simulink model "w2_warplab_agc"  (Simulink 7.7)
settings: Solver=ode45  StartTime=0.0  StopTime=2e5  RelTol=1e-3
PostLoadFcn:
  | w2_warplab_agc_init
InitFcn:
  | w2_warplab_agc_init
StartFcn:
  | w2_warplab_agc_init
values from neighbouring files (symbols this model uses):
  PHY_CONFIG_PKT_DET_CORR_THRESH = 90    [w2_warplab_agc_init.m]
  PHY_CONFIG_PKT_DET_ENERGY_THRESH = 14    [w2_warplab_agc_init.m]
  PHY_CONFIG_PKT_DET_MIN_DURR = 4    [w2_warplab_agc_init.m]
undefined symbols (not defined in the file or in its folder): gcbh, xlBlockLoadCallback, xlGetNormalizedPeriod
libraries: xbsIndex_r4 x1000, simulink x1
(part 2 of 7)

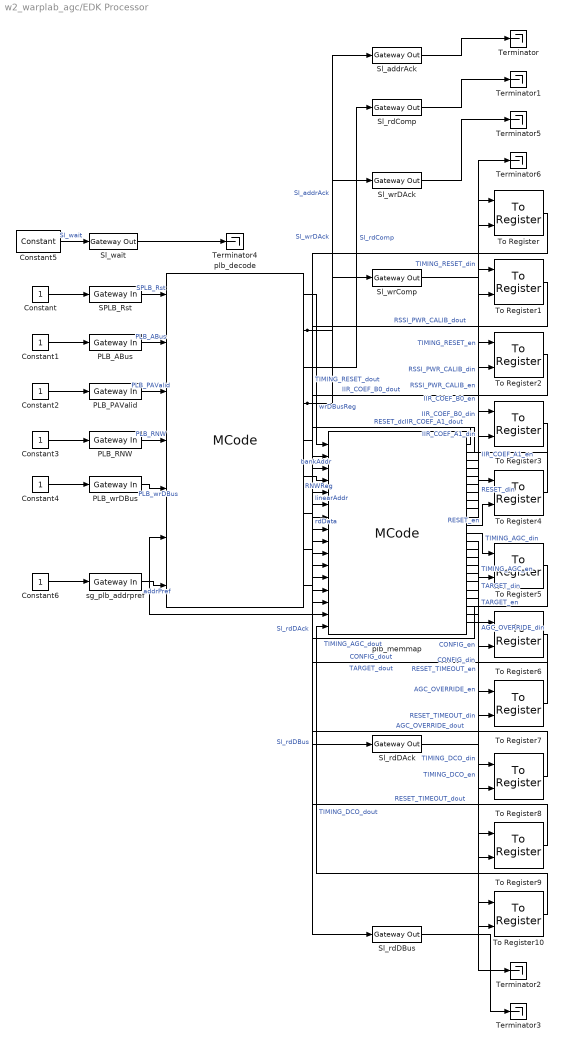
== system w2_warplab_agc/EDK Processor ==
  Constant{,1..4,6} (6 alike) : Constant
  Constant5 : xbsIndex_r4/Constant  const=0  gui_display_data_type=Fixed-point  arith_type=Unsigned  n_bits=1  bin_pt=0  preci_type=Single  exp_width=8  frac_width=24  explicit_period=on  period=xlGetNormalizedPeriod()  equ=P=C  opselect=C  inp2=PCIN>>17  opr=+  inp1=P  carry=CIN  dbl_ovrd=off  block_type=constant
  PLB_ABus : xbsIndex_r4/Gateway In  gui_display_data_type=Fixed-point  arith_type=Unsigned  n_bits=32  bin_pt=0  preci_type=Single  exp_width=8  frac_width=24  quantization="Round  (unbiased: +/- Inf)"  overflow=Saturate  period=xlGetNormalizedPeriod()  dbl_ovrd=off  timing_constraint=None  locs_specified=off  LOCs={}  UseAsADC=off  ADCChannel='1'  inherit_from_input=off  hdl_port=on  block_type=gatewayin
      settings: sginterface={'Xilinx'=>{'jtaghwcosim'=>{'non_memory_mapped_port'=>'PLB_ABus'}},'iopad'=>{'constraint'=>'#'}}
  PLB_PAValid : xbsIndex_r4/Gateway In  gui_display_data_type=Fixed-point  arith_type=Unsigned  n_bits=1  bin_pt=0  preci_type=Single  exp_width=8  frac_width=24  quantization="Round  (unbiased: +/- Inf)"  overflow=Saturate  period=xlGetNormalizedPeriod()  dbl_ovrd=off  timing_constraint=None  locs_specified=off  LOCs={}  UseAsADC=off  ADCChannel='1'  inherit_from_input=off  hdl_port=on  block_type=gatewayin
      settings: sginterface={'Xilinx'=>{'jtaghwcosim'=>{'non_memory_mapped_port'=>'PLB_PAValid'}},'iopad'=>{'constraint'=>'#'}}
  PLB_RNW : xbsIndex_r4/Gateway In  gui_display_data_type=Fixed-point  arith_type=Unsigned  n_bits=1  bin_pt=0  preci_type=Single  exp_width=8  frac_width=24  quantization="Round  (unbiased: +/- Inf)"  overflow=Saturate  period=xlGetNormalizedPeriod()  dbl_ovrd=off  timing_constraint=None  locs_specified=off  LOCs={}  UseAsADC=off  ADCChannel='1'  inherit_from_input=off  hdl_port=on  block_type=gatewayin
      settings: sginterface={'Xilinx'=>{'jtaghwcosim'=>{'non_memory_mapped_port'=>'PLB_RNW'}},'iopad'=>{'constraint'=>'#'}}
  PLB_wrDBus : xbsIndex_r4/Gateway In  gui_display_data_type=Fixed-point  arith_type=Unsigned  n_bits=32  bin_pt=0  preci_type=Single  exp_width=8  frac_width=24  quantization="Round  (unbiased: +/- Inf)"  overflow=Saturate  period=xlGetNormalizedPeriod()  dbl_ovrd=off  timing_constraint=None  locs_specified=off  LOCs={}  UseAsADC=off  ADCChannel='1'  inherit_from_input=off  hdl_port=on  block_type=gatewayin
      settings: sginterface={'Xilinx'=>{'jtaghwcosim'=>{'non_memory_mapped_port'=>'PLB_wrDBus'}},'iopad'=>{'constraint'=>'#'}}
  SPLB_Rst : xbsIndex_r4/Gateway In  gui_display_data_type=Fixed-point  arith_type=Unsigned  n_bits=1  bin_pt=0  preci_type=Single  exp_width=8  frac_width=24  quantization="Round  (unbiased: +/- Inf)"  overflow=Saturate  period=xlGetNormalizedPeriod()  dbl_ovrd=off  timing_constraint=None  locs_specified=off  LOCs={}  UseAsADC=off  ADCChannel='1'  inherit_from_input=off  hdl_port=on  block_type=gatewayin
      settings: sginterface={'Xilinx'=>{'jtaghwcosim'=>{'non_memory_mapped_port'=>'SPLB_Rst'}},'iopad'=>{'constraint'=>'#'}}
  Sl_addrAck : xbsIndex_r4/Gateway Out  inherit_from_input=off  hdl_port=on  timing_constraint=None  locs_specified=off  LOCs={}  UseAsDAC=off  DACChannel='1'  block_type=gatewayout
      settings: sginterface={'Xilinx'=>{'jtaghwcosim'=>{'non_memory_mapped_port'=>'Sl_addrAck'}},'iopad'=>{'constraint'=>'#'}}
  Sl_rdComp : xbsIndex_r4/Gateway Out  inherit_from_input=off  hdl_port=on  timing_constraint=None  locs_specified=off  LOCs={}  UseAsDAC=off  DACChannel='1'  block_type=gatewayout
      settings: sginterface={'Xilinx'=>{'jtaghwcosim'=>{'non_memory_mapped_port'=>'Sl_rdComp'}},'iopad'=>{'constraint'=>'#'}}
  Sl_rdDAck : xbsIndex_r4/Gateway Out  inherit_from_input=off  hdl_port=on  timing_constraint=None  locs_specified=off  LOCs={}  UseAsDAC=off  DACChannel='1'  block_type=gatewayout
      settings: sginterface={'Xilinx'=>{'jtaghwcosim'=>{'non_memory_mapped_port'=>'Sl_rdDAck'}},'iopad'=>{'constraint'=>'#'}}
  Sl_rdDBus : xbsIndex_r4/Gateway Out  inherit_from_input=off  hdl_port=on  timing_constraint=None  locs_specified=off  LOCs={}  UseAsDAC=off  DACChannel='1'  block_type=gatewayout
      settings: sginterface={'Xilinx'=>{'jtaghwcosim'=>{'non_memory_mapped_port'=>'Sl_rdDBus'}},'iopad'=>{'constraint'=>'#'}}
  Sl_wait : xbsIndex_r4/Gateway Out  inherit_from_input=off  hdl_port=on  timing_constraint=None  locs_specified=off  LOCs={}  UseAsDAC=off  DACChannel='1'  block_type=gatewayout
      settings: sginterface={'Xilinx'=>{'jtaghwcosim'=>{'non_memory_mapped_port'=>'Sl_wait'}},'iopad'=>{'constraint'=>'#'}}
  Sl_wrComp : xbsIndex_r4/Gateway Out  inherit_from_input=off  hdl_port=on  timing_constraint=None  locs_specified=off  LOCs={}  UseAsDAC=off  DACChannel='1'  block_type=gatewayout
      settings: sginterface={'Xilinx'=>{'jtaghwcosim'=>{'non_memory_mapped_port'=>'Sl_wrComp'}},'iopad'=>{'constraint'=>'#'}}
  Sl_wrDAck : xbsIndex_r4/Gateway Out  inherit_from_input=off  hdl_port=on  timing_constraint=None  locs_specified=off  LOCs={}  UseAsDAC=off  DACChannel='1'  block_type=gatewayout
      settings: sginterface={'Xilinx'=>{'jtaghwcosim'=>{'non_memory_mapped_port'=>'Sl_wrDAck'}},'iopad'=>{'constraint'=>'#'}}
  Terminator{,1..6} (7 alike) : Terminator
  To Register : xbsIndex_r4/To Register  shared_memory_name='TIMING_RESET'  init=0  ownership=Owned and initialized elsewhere  explicit_data_type=on  gui_display_data_type=Fixed-point  arith_type=Unsigned  n_bits=32  bin_pt=0  preci_type=Single  dbl_ovrd=off  block_type=toreg
      settings: AttributesFormatString=<< %<shared_memory_name> >>  infoedit="Register block that writes data to a shared memory register.  Delay of one sample period."
  To Register1 : xbsIndex_r4/To Register  shared_memory_name='RSSI_PWR_CALIB'  init=0  ownership=Owned and initialized elsewhere  explicit_data_type=on  gui_display_data_type=Fixed-point  arith_type=Unsigned  n_bits=32  bin_pt=0  preci_type=Single  dbl_ovrd=off  block_type=toreg
      settings: AttributesFormatString=<< %<shared_memory_name> >>  infoedit="Register block that writes data to a shared memory register.  Delay of one sample period."
  To Register10 : xbsIndex_r4/To Register  shared_memory_name='TIMING_DCO'  init=0  ownership=Owned and initialized elsewhere  explicit_data_type=on  gui_display_data_type=Fixed-point  arith_type=Unsigned  n_bits=32  bin_pt=0  preci_type=Single  dbl_ovrd=off  block_type=toreg
      settings: AttributesFormatString=<< %<shared_memory_name> >>  infoedit="Register block that writes data to a shared memory register.  Delay of one sample period."
  To Register2 : xbsIndex_r4/To Register  shared_memory_name='IIR_COEF_B0'  init=0  ownership=Owned and initialized elsewhere  explicit_data_type=on  gui_display_data_type=Fixed-point  arith_type=Unsigned  n_bits=18  bin_pt=17  preci_type=Single  dbl_ovrd=off  block_type=toreg
      settings: AttributesFormatString=<< %<shared_memory_name> >>  infoedit="Register block that writes data to a shared memory register.  Delay of one sample period."
  To Register3 : xbsIndex_r4/To Register  shared_memory_name='IIR_COEF_A1'  init=0  ownership=Owned and initialized elsewhere  explicit_data_type=on  gui_display_data_type=Fixed-point  arith_type="Signed  (2's comp)"  n_bits=18  bin_pt=17  preci_type=Single  dbl_ovrd=off  block_type=toreg
      settings: AttributesFormatString=<< %<shared_memory_name> >>  infoedit="Register block that writes data to a shared memory register.  Delay of one sample period."
  To Register4 : xbsIndex_r4/To Register  shared_memory_name='RESET'  init=0  ownership=Owned and initialized elsewhere  explicit_data_type=on  gui_display_data_type=Fixed-point  arith_type=Unsigned  n_bits=32  bin_pt=0  preci_type=Single  dbl_ovrd=off  block_type=toreg
      settings: AttributesFormatString=<< %<shared_memory_name> >>  infoedit="Register block that writes data to a shared memory register.  Delay of one sample period."
  To Register5 : xbsIndex_r4/To Register  shared_memory_name='TIMING_AGC'  init=0  ownership=Owned and initialized elsewhere  explicit_data_type=on  gui_display_data_type=Fixed-point  arith_type=Unsigned  n_bits=32  bin_pt=0  preci_type=Single  dbl_ovrd=off  block_type=toreg
      settings: AttributesFormatString=<< %<shared_memory_name> >>  infoedit="Register block that writes data to a shared memory register.  Delay of one sample period."
  To Register6 : xbsIndex_r4/To Register  shared_memory_name='TARGET'  init=0  ownership=Owned and initialized elsewhere  explicit_data_type=on  gui_display_data_type=Fixed-point  arith_type=Unsigned  n_bits=32  bin_pt=0  preci_type=Single  dbl_ovrd=off  block_type=toreg
      settings: AttributesFormatString=<< %<shared_memory_name> >>  infoedit="Register block that writes data to a shared memory register.  Delay of one sample period."
  To Register7 : xbsIndex_r4/To Register  shared_memory_name='CONFIG'  init=0  ownership=Owned and initialized elsewhere  explicit_data_type=on  gui_display_data_type=Fixed-point  arith_type=Unsigned  n_bits=32  bin_pt=0  preci_type=Single  dbl_ovrd=off  block_type=toreg
      settings: AttributesFormatString=<< %<shared_memory_name> >>  infoedit="Register block that writes data to a shared memory register.  Delay of one sample period."
  To Register8 : xbsIndex_r4/To Register  shared_memory_name='AGC_OVERRIDE'  init=0  ownership=Owned and initialized elsewhere  explicit_data_type=on  gui_display_data_type=Fixed-point  arith_type=Unsigned  n_bits=32  bin_pt=0  preci_type=Single  dbl_ovrd=off  block_type=toreg
      settings: AttributesFormatString=<< %<shared_memory_name> >>  infoedit="Register block that writes data to a shared memory register.  Delay of one sample period."
  To Register9 : xbsIndex_r4/To Register  shared_memory_name='RESET_TIMEOUT'  init=0  ownership=Owned and initialized elsewhere  explicit_data_type=on  gui_display_data_type=Fixed-point  arith_type=Unsigned  n_bits=32  bin_pt=0  preci_type=Single  dbl_ovrd=off  block_type=toreg
      settings: AttributesFormatString=<< %<shared_memory_name> >>  infoedit="Register block that writes data to a shared memory register.  Delay of one sample period."
  plb_decode : xbsIndex_r4/MCode  mfname=xlmax  explicit_period=off  period=1  dbl_ovrd=off  enable_stdout=off  enable_debug=off  mfilecontent=|  suppress_output=on  defparams={}  hide_port_list={}  block_type=mcode
      | function [wrDBusReg, addrAck, rdComp, wrDAck, bankAddr, RNWReg, rdDAck, rdDBus, linearAddr] = plb_bus_decode(plbRst, plbABus, plbPAValid, plbRNW, plbWrDBus, rdData, addrPref)
      | 
      | % constant variables (TODO: should pass from outside)
      | ADDRPREF_LEN = 20;
      | BANKADDR_LEN = 2;
      | LINEARADDR_LEN = 8;
      | ABUS_LEN = 32;
      | DBUS_LEN = 32;
      | 
      | % declare and initialize persistent variables
      | % register input bus signals
      | persistent plbRstReg_, plbRstReg_ = xl_state(0, {xlBoolean});
      | persistent plbABusReg_, plbABusReg_ = xl_state(0, {xlUnsigned, ABUS_LEN, 0});
      | persistent plbPAValidReg_, plbPAValidReg_ = xl_state(0, {xlBoolean});
      | persistent plbRNWReg_, plbRNWReg_ = xl_state(0, {xlUnsigned, 1, 0});
      | persistent plbWrDBusReg_, plbWrDBusReg_ = xl_state(0, {xlUnsigned, DBUS_LEN, 0});
      | 
      | % ===== rest of the outputs =====
      | 
      | bankAddr   = xl_slice(plbABusReg_, 2+BANKADDR_LEN+LINEARADDR_LEN-1, 2+LINEARADDR_LEN);
      | linearAddr = xl_slice(plbABusReg_, 2+LINEARADDR_LEN-1, 2);
      | RNWReg = plbRNWReg_;
      | wrDBusReg = plbWrDBusReg_;
      | 
      | % ===== p_select =====
      | 
      | % register PAValid
      | persistent aValidReg, aValidReg = xl_state(0, {xlBoolean});
      | aValidReg = plbPAValidReg_;
      | 
      | % extract and register the address prefix
      | addrPref_in = xl_slice(plbABusReg_, xl_nbits(plbABusReg_)-1, xl_nbits(plbABusReg_)-ADDRPREF_LEN);
      | if addrPref_in == addrPref
      |     ps1 = true;
      | else 
      |     ps1 = false;
      | end 
      | 
      | persistent ps1Reg, ps1Reg = xl_state(0, ps1);
      | ps1Reg = ps1;
      | 
      | ps = xl_and(ps1Reg, aValidReg);
      | 
      | % ===== addrAck =====
      | 
      | % register ps
      | persistent psReg, psReg = xl_state(0, ps);
      | 
      | addrAck = xfix({xlUnsigned, 1, 0}, xl_and(xl_not(plbRstReg_), ps, xl_not(psReg)));
      | 
      | psReg = ps;
      | 
      | % ===== rdComp, rd/wr DAck =====
      |  
      | rdComp1 = xfix({xlUnsigned, 1, 0}, xl_and(addrAck, RNWReg));
      | 
      | NUM_rdCompDelay = 3;
      | persistent rdCompDelay, rdCompDelay = xl_state(zeros(1, NUM_rdCompDelay), rdComp1, NUM_rdCompDelay);
      | rdComp2 = rdCompDelay.back;
      | rdCompDelay.push_front_pop_back(rdComp1);
      | 
      | persistent rdCompReg, rdCompReg = xl_state(0, rdComp1);
      | rdComp = rdCompReg;
      | rdCompReg = rdComp2;
      | 
      | persistent rdDAckReg, rdDAckReg = xl_state(0, rdComp1);
      | rdDAck = rdDAckReg;
      | rdDAckReg = rdComp;
      | 
      | persistent wrDAckReg, wrDAckReg = xl_state(0, addrAck);
      | wrDAck = wrDAckReg;
      | wrDAckReg = xl_and(addrAck, xl_not(RNWReg));
      | 
      | % ===== rdDBus =====
      | 
      | rdSel = xl_or(rdComp2, rdComp);
      | 
      | if rdSel == 1
      |     rdDBus1 = rdData;
      | else
      |     rdDBus1 = 0;
      | end % if
      | 
      | persistent rdDBusReg, rdDBusReg = xl_state(0, rdDBus1);
      | rdDBus = rdDBusReg;
      | rdDBusReg = rdDBus1;
      | 
      | % rdDBus = xl_concat(rdDBus32, rdDBus32);
      | % rdDBus = rdDBus32;
      | 
      | % ===== update the persistent variables =====
      | 
      | plbRstReg_ = plbRst;
      | plbABusReg_ = plbABus;
      | plbPAValidReg_ = plbPAValid;
      | plbRNWReg_ = plbRNW;
      | plbWrDBusReg_ = xl_slice(plbWrDBus, DBUS_LEN-1, 0);
  plb_memmap : xbsIndex_r4/MCode  mfname=xlmax  explicit_period=off  period=1  dbl_ovrd=off  enable_stdout=off  enable_debug=off  mfilecontent=|  suppress_output=on  defparams={}  hide_port_list={}  block_type=mcode
      | function [read_bank_out, sm_TIMING_RESET_din, sm_TIMING_RESET_en, sm_RSSI_PWR_CALIB_din, sm_RSSI_PWR_CALIB_en, sm_IIR_COEF_B0_din, sm_IIR_COEF_B0_en, sm_IIR_COEF_A1_din, sm_IIR_COEF_A1_en, sm_RESET_din, sm_RESET_en, sm_TIMING_AGC_din, sm_TIMING_AGC_en, sm_TARGET_din, sm_TARGET_en, sm_CONFIG_din, sm_CONFIG_en, sm_AGC_OVERRIDE_din, sm_AGC_OVERRIDE_en, sm_RESET_TIMEOUT_din, sm_RESET_TIMEOUT_en, sm_TIMING_DCO_din, sm_TIMING_DCO_en] = plb_memmap(wrDBus, bankAddr, linearAddr, RNWReg, addrAck, sm_TIMING_RESET, sm_RSSI_PWR_CALIB, sm_IIR_COEF_B0, sm_IIR_COEF_A1, sm_RESET, sm_TIMING_AGC, sm_TARGET, sm_CONFIG, sm_AGC_OVERRIDE, sm_RESET_TIMEOUT, sm_TIMING_DCO)
      | 
      | 
      | % connvert the input data to UFix_32_0 (the bus data type)
      | % 'From Register' blocks
      | % 'To Register' blocks
      | 
      | % sm_TIMING_RESET_dout = xfix({xlUnsigned, 32, 0}, 0);
      | sm_TIMING_RESET_dout = xl_force(sm_TIMING_RESET, xlUnsigned, 0);
      | 
      | % sm_RSSI_PWR_CALIB_dout = xfix({xlUnsigned, 32, 0}, 0);
      | sm_RSSI_PWR_CALIB_dout = xl_force(sm_RSSI_PWR_CALIB, xlUnsigned, 0);
      | 
      | % sm_IIR_COEF_B0_dout = xfix({xlUnsigned, 32, 0}, 0);
      | sm_IIR_COEF_B0_dout = xl_force(sm_IIR_COEF_B0, xlUnsigned, 0);
      | 
      | % sm_IIR_COEF_A1_dout = xfix({xlUnsigned, 32, 0}, 0);
      | sm_IIR_COEF_A1_dout = xl_force(sm_IIR_COEF_A1, xlUnsigned, 0);
      | 
      | % sm_RESET_dout = xfix({xlUnsigned, 32, 0}, 0);
      | sm_RESET_dout = xl_force(sm_RESET, xlUnsigned, 0);
      | 
      | % sm_TIMING_AGC_dout = xfix({xlUnsigned, 32, 0}, 0);
      | sm_TIMING_AGC_dout = xl_force(sm_TIMING_AGC, xlUnsigned, 0);
      | 
      | % sm_TARGET_dout = xfix({xlUnsigned, 32, 0}, 0);
      | sm_TARGET_dout = xl_force(sm_TARGET, xlUnsigned, 0);
      | 
      | % sm_CONFIG_dout = xfix({xlUnsigned, 32, 0}, 0);
      | sm_CONFIG_dout = xl_force(sm_CONFIG, xlUnsigned, 0);
      | 
      | % sm_AGC_OVERRIDE_dout = xfix({xlUnsigned, 32, 0}, 0);
      | sm_AGC_OVERRIDE_dout = xl_force(sm_AGC_OVERRIDE, xlUnsigned, 0);
      | 
      | % sm_RESET_TIMEOUT_dout = xfix({xlUnsigned, 32, 0}, 0);
      | sm_RESET_TIMEOUT_dout = xl_force(sm_RESET_TIMEOUT, xlUnsigned, 0);
      | 
      | % sm_TIMING_DCO_dout = xfix({xlUnsigned, 32, 0}, 0);
      | sm_TIMING_DCO_dout = xl_force(sm_TIMING_DCO, xlUnsigned, 0);
      | 
      | 
      | % 'From FIFO' blocks
      | % 'To FIFO' blocks
      | % 'Shared Memory' blocks
      | 
      | % 'dout' ports of 'From Register' blocks
      | 
      | % registered register mux output
      | persistent reg_bank_out_reg; reg_bank_out_reg = xl_state(0, {xlUnsigned, 32, 0});
      | reg_bank_out = reg_bank_out_reg;
      | 
      | if linearAddr == 0
      |     reg_bank_out_reg = sm_TIMING_RESET_dout;
      | elseif linearAddr == 1
      |     reg_bank_out_reg = sm_RSSI_PWR_CALIB_dout;
      | elseif linearAddr == 2
      |     reg_bank_out_reg = sm_IIR_COEF_B0_dout;
      | elseif linearAddr == 3
      |     reg_bank_out_reg = sm_IIR_COEF_A1_dout;
      | elseif linearAddr == 4
      |     reg_bank_out_reg = sm_RESET_dout;
      | elseif linearAddr == 5
      |     reg_bank_out_reg = sm_TIMING_AGC_dout;
      | elseif linearAddr == 6
      |     reg_bank_out_reg = sm_TARGET_dout;
      | elseif linearAddr == 7
      |     reg_bank_out_reg = sm_CONFIG_dout;
      | elseif linearAddr == 8
      |     reg_bank_out_reg = sm_AGC_OVERRIDE_dout;
      | elseif linearAddr == 9
      |     reg_bank_out_reg = sm_RESET_TIMEOUT_dout;
      | elseif linearAddr == 10
      |     reg_bank_out_reg = sm_TIMING_DCO_dout;
      | 
      | end
      | 
      | 
      | % 'From FIFO' and 'To FIFO' blocks
      | 
      | 
      | 
      | 
      | 
      | opCode = xl_concat(addrAck, RNWReg, bankAddr, linearAddr);
      | 
      | % 'Shared Memory' blocks
      | 
      | 
      | 
      | 
      | 
      | % 'din' ports of 'Shared Memory' blocks
      | 
      | 
      | % 'we' ports of 'Shared Memory' blocks
      | 
      | 
      | % 'addr' ports of 'Shared Memory' blocks
      | 
      | 
      | % 're' ports of 'From FIFO' blocks
      | 
      | 
      | % 'en' ports of 'To Register' blocks
      | if opCode == xl_concat(xfix({xlUnsigned, 4, 0}, 10), ...
      |                        xfix({xlUnsigned, xl_nbits(linearAddr), 0}, 0))
      |     sm_TIMING_RESET_en = true;
      | else
      |     sm_TIMING_RESET_en = false;
      | end
      | if opCode == xl_concat(xfix({xlUnsigned, 4, 0}, 10), ...
      |                        xfix({xlUnsigned, xl_nbits(linearAddr), 0}, 1))
      |     sm_RSSI_PWR_CALIB_en = true;
      | else
      |     sm_RSSI_PWR_CALIB_en = false;
      | end
      | if opCode == xl_concat(xfix({xlUnsigned, 4, 0}, 10), ...
      |                        xfix({xlUnsigned, xl_nbits(linearAddr), 0}, 2))
      |     sm_IIR_COEF_B0_en = true;
      | else
      |     sm_IIR_COEF_B0_en = false;
      | end
      | if opCode == xl_concat(xfix({xlUnsigned, 4, 0}, 10), ...
      |                        xfix({xlUnsigned, xl_nbits(linearAddr), 0}, 3))
      |     sm_IIR_COEF_A1_en = true;
      | else
      |     sm_IIR_COEF_A1_en = false;
      | end
      | if opCode == xl_concat(xfix({xlUnsigned, 4, 0}, 10), ...
      |                        xfix({xlUnsigned, xl_nbits(linearAddr), 0}, 4))
      |     sm_RESET_en = true;
      | else
      |     sm_RESET_en = false;
      | end
      | if opCode == xl_concat(xfix({xlUnsigned, 4, 0}, 10), ...
      |                        xfix({xlUnsigned, xl_nbits(linearAddr), 0}, 5))
      |     sm_TIMING_AGC_en = true;
      | else
      |     sm_TIMING_AGC_en = false;
      | end
      | if opCode == xl_concat(xfix({xlUnsigned, 4, 0}, 10), ...
      |                        xfix({xlUnsigned, xl_nbits(linearAddr), 0}, 6))
      |     sm_TARGET_en = true;
      | else
      |     sm_TARGET_en = false;
      | end
      | if opCode == xl_concat(xfix({xlUnsigned, 4, 0}, 10), ...
      |                        xfix({xlUnsigned, xl_nbits(linearAddr), 0}, 7))
      |     sm_CONFIG_en = true;
      | else
      |     sm_CONFIG_en = false;
      | end
      | if opCode == xl_concat(xfix({xlUnsigned, 4, 0}, 10), ...
      |                        xfix({xlUnsigned, xl_nbits(linearAddr), 0}, 8))
      |     sm_AGC_OVERRIDE_en = true;
      | else
      |     sm_AGC_OVERRIDE_en = false;
      | end
      | if opCode == xl_concat(xfix({xlUnsigned, 4, 0}, 10), ...
      |                        xfix({xlUnsigned, xl_nbits(linearAddr), 0}, 9))
      |     sm_RESET_TIMEOUT_en = true;
      | else
      |     sm_RESET_TIMEOUT_en = false;
      | end
      | if opCode == xl_concat(xfix({xlUnsigned, 4, 0}, 10), ...
      |                        xfix({xlUnsigned, xl_nbits(linearAddr), 0}, 10))
      |     sm_TIMING_DCO_en = true;
      | else
      |     sm_TIMING_DCO_en = false;
      | end
      | 
      | 
      | % 'din' ports of 'To FIFO' blocks
      | 
      | 
      | % 'we' ports of 'To FIFO' blocks
      | 
      | 
      | % 'din' ports of 'To Register' blocks
      | sm_TIMING_RESET_din = xl_force(xl_slice(wrDBus, 32 - 1, 0), ...
      |                                  xlUnsigned, ...
      |                                  0);
      | sm_RSSI_PWR_CALIB_din = xl_force(xl_slice(wrDBus, 32 - 1, 0), ...
      |                                  xlUnsigned, ...
      |                                  0);
      | sm_IIR_COEF_B0_din = xl_force(xl_slice(wrDBus, 18 - 1, 0), ...
      |                                  xlUnsigned, ...
      |                                  17);
      | sm_IIR_COEF_A1_din = xl_force(xl_slice(wrDBus, 18 - 1, 0), ...
      |                                  xlSigned, ...
      |                                  17);
      | sm_RESET_din = xl_force(xl_slice(wrDBus, 32 - 1, 0), ...
      |                                  xlUnsigned, ...
      |                                  0);
      | sm_TIMING_AGC_din = xl_force(xl_slice(wrDBus, 32 - 1, 0), ...
      |                                  xlUnsigned, ...
      |                                  0);
      | sm_TARGET_din = xl_force(xl_slice(wrDBus, 32 - 1, 0), ...
      |                                  xlUnsigned, ...
      |                                  0);
      | sm_CONFIG_din = xl_force(xl_slice(wrDBus, 32 - 1, 0), ...
      |                                  xlUnsigned, ...
      |                                  0);
      | sm_AGC_OVERRIDE_din = xl_force(xl_slice(wrDBus, 32 - 1, 0), ...
      |                                  xlUnsigned, ...
      |                                  0);
      | sm_RESET_TIMEOUT_din = xl_force(xl_slice(wrDBus, 32 - 1, 0), ...
      |                                  xlUnsigned, ...
      |                                  0);
      | sm_TIMING_DCO_din = xl_force(xl_slice(wrDBus, 32 - 1, 0), ...
      |                                  xlUnsigned, ...
      |                                  0);
      | 
      | 
      | persistent read_bank_out_reg; read_bank_out_reg = xl_state(0, {xlUnsigned, 32, 0});
      | read_bank_out = read_bank_out_reg;
      | 
      | persistent bankAddr_reg; bankAddr_reg = xl_state(0, bankAddr);
      | 
      | if bankAddr_reg == 0
      |     % Bank 0: Shared Memories
      |     read_bank_out_reg = 0;
      | elseif bankAddr_reg == 1
      |     % Bank 1: From/To FIFOs
      |     read_bank_out_reg =  0;
      | elseif bankAddr_reg == 2
      |     % Bank 2: From/To Registers
      |     read_bank_out_reg = reg_bank_out;
      | elseif bankAddr_reg == 3
      |     % Bank 3: Configuration Registers
      |     read_bank_out_reg = 0;
      | end
      | 
      | bankAddr_reg = bankAddr;
  sg_plb_addrpref : xbsIndex_r4/Gateway In  gui_display_data_type=Fixed-point  arith_type=Unsigned  n_bits=20  bin_pt=0  preci_type=Single  exp_width=8  frac_width=24  quantization="Round  (unbiased: +/- Inf)"  overflow=Saturate  period=xlGetNormalizedPeriod()  dbl_ovrd=off  timing_constraint=None  locs_specified=off  LOCs={}  UseAsADC=off  ADCChannel='1'  inherit_from_input=off  hdl_port=on  block_type=gatewayin
      settings: sginterface={'Xilinx'=>{'jtaghwcosim'=>{'non_memory_mapped_port'=>'sg_plb_addrpref'}},'iopad'=>{'constraint'=>'#'}}
  wires:
  plb_decode/2 -> plb_memmap/5, Sl_addrAck/1  "Sl_addrAck"
  plb_decode/4 -> Sl_wrDAck/1, Sl_wrComp/1  "Sl_wrDAck"
  plb_memmap/23 -> To Register10/2  "TIMING_DCO_en"
  plb_memmap/22 -> To Register10/1  "TIMING_DCO_din"
  plb_memmap/21 -> To Register9/2  "RESET_TIMEOUT_en"
  plb_memmap/20 -> To Register9/1  "RESET_TIMEOUT_din"
  plb_memmap/19 -> To Register8/2  "AGC_OVERRIDE_en"
  plb_memmap/18 -> To Register8/1  "AGC_OVERRIDE_din"
  plb_memmap/17 -> To Register7/2  "CONFIG_en"
  plb_memmap/16 -> To Register7/1  "CONFIG_din"
  plb_memmap/15 -> To Register6/2  "TARGET_en"
  plb_memmap/14 -> To Register6/1  "TARGET_din"
  plb_memmap/13 -> To Register5/2  "TIMING_AGC_en"
  plb_memmap/12 -> To Register5/1  "TIMING_AGC_din"
  plb_memmap/11 -> To Register4/2  "RESET_en"
  plb_memmap/10 -> To Register4/1  "RESET_din"
  plb_memmap/9 -> To Register3/2  "IIR_COEF_A1_en"
  plb_memmap/8 -> To Register3/1  "IIR_COEF_A1_din"
  plb_memmap/7 -> To Register2/2  "IIR_COEF_B0_en"
  plb_memmap/6 -> To Register2/1  "IIR_COEF_B0_din"
  plb_memmap/5 -> To Register1/2  "RSSI_PWR_CALIB_en"
  plb_memmap/4 -> To Register1/1  "RSSI_PWR_CALIB_din"
  plb_memmap/3 -> To Register/2  "TIMING_RESET_en"
  plb_memmap/2 -> To Register/1  "TIMING_RESET_din"
  plb_memmap/1 -> plb_decode/6  "rdData"
  To Register10/1 -> plb_memmap/16  "TIMING_DCO_dout"
  To Register9/1 -> plb_memmap/15  "RESET_TIMEOUT_dout"
  To Register8/1 -> plb_memmap/14  "AGC_OVERRIDE_dout"
  To Register7/1 -> plb_memmap/13  "CONFIG_dout"
  To Register6/1 -> plb_memmap/12  "TARGET_dout"
  To Register5/1 -> plb_memmap/11  "TIMING_AGC_dout"
  To Register4/1 -> plb_memmap/10  "RESET_dout"
  To Register3/1 -> plb_memmap/9  "IIR_COEF_A1_dout"
  To Register2/1 -> plb_memmap/8  "IIR_COEF_B0_dout"
  To Register1/1 -> plb_memmap/7  "RSSI_PWR_CALIB_dout"
  To Register/1 -> plb_memmap/6  "TIMING_RESET_dout"
  plb_decode/6 -> plb_memmap/4  "RNWReg"
  plb_decode/9 -> plb_memmap/3  "linearAddr"
  plb_decode/5 -> plb_memmap/2  "bankAddr"
  plb_decode/1 -> plb_memmap/1  "wrDBusReg"
  plb_decode/8 -> Sl_rdDBus/1  "Sl_rdDBus"
  plb_decode/7 -> Sl_rdDAck/1  "Sl_rdDAck"
  plb_decode/3 -> Sl_rdComp/1  "Sl_rdComp"
  sg_plb_addrpref/1 -> plb_decode/7  "addrPref"
  PLB_wrDBus/1 -> plb_decode/5  "PLB_wrDBus"
  PLB_RNW/1 -> plb_decode/4  "PLB_RNW"
  PLB_PAValid/1 -> plb_decode/3  "PLB_PAValid"
  PLB_ABus/1 -> plb_decode/2  "PLB_ABus"
  SPLB_Rst/1 -> plb_decode/1  "SPLB_Rst"
  Constant6/1 -> sg_plb_addrpref/1
  Constant5/1 -> Sl_wait/1  "Sl_wait"
  Constant4/1 -> PLB_wrDBus/1
  Constant3/1 -> PLB_RNW/1
  Constant2/1 -> PLB_PAValid/1
  Constant1/1 -> PLB_ABus/1
  Constant/1 -> SPLB_Rst/1
  Sl_wrComp/1 -> Terminator6/1
  Sl_wrDAck/1 -> Terminator5/1
  Sl_wait/1 -> Terminator4/1
  Sl_rdDBus/1 -> Terminator3/1
  Sl_rdDAck/1 -> Terminator2/1
  Sl_rdComp/1 -> Terminator1/1
  Sl_addrAck/1 -> Terminator/1

== system w2_warplab_agc/Gain Calc A ==
  I : Inport
  Q : Inport  Port=2
  IQ Valid : Inport  Port=3
  RSSI : Inport  Port=4
  BB gain : Subsystem
  Capture & Convert : Subsystem
  IQ Mag : Subsystem
  RF Gain : Subsystem
  RSSI Avg : Subsystem
  Register{1..4} (4 alike) : xbsIndex_r4/Register  init=0  rst=off  en=off  dbl_ovrd=off  block_type=register
  G_RF : Outport
  G_BB : Outport  Port=2
  wires:
  RF Gain/1(G_RF) -> Register1/1, Capture & Convert/1(G_RF)
  Register1/1 -> Register2/1
  RSSI/1 -> RSSI Avg/1(RSSI)
  RSSI Avg/1(avg) -> Capture & Convert/2(RSSI)
  Capture & Convert/1(Rx Pwr (dBm)) -> RF Gain/1(Rx Pwr), BB gain/2(P_IN_RSSI)
  Register3/1 -> Register4/1
  BB gain/1(G_BB) -> Register3/1
  RF Gain/2(G_RF_dB) -> BB gain/1(G_RF_dB)
  IQ Mag/1(IQ_dBv) -> BB gain/3(IQ_dBv)
  I/1 -> IQ Mag/1(I)
  Q/1 -> IQ Mag/2(Q)
  IQ Valid/1 -> IQ Mag/3(Valid)
  Register2/1 -> G_RF/1
  Register4/1 -> G_BB/1

== system w2_warplab_agc/Gain Calc B ==
  I : Inport
  Q : Inport  Port=2
  IQ Valid : Inport  Port=3
  RSSI : Inport  Port=4
  BB gain : Subsystem
  Capture & Convert : Subsystem
  IQ Mag : Subsystem
  RF Gain : Subsystem
  RSSI Avg : Subsystem
  Register{1..4} (4 alike) : xbsIndex_r4/Register  init=0  rst=off  en=off  dbl_ovrd=off  block_type=register
  G_RF : Outport
  G_BB : Outport  Port=2
  wires:
  Register4/1 -> G_BB/1
  Register2/1 -> G_RF/1
  IQ Valid/1 -> IQ Mag/3(Valid)
  Q/1 -> IQ Mag/2(Q)
  I/1 -> IQ Mag/1(I)
  IQ Mag/1(IQ_dBv) -> BB gain/3(IQ_dBv)
  RF Gain/2(G_RF_dB) -> BB gain/1(G_RF_dB)
  BB gain/1(G_BB) -> Register3/1
  Register3/1 -> Register4/1
  Capture & Convert/1(Rx Pwr (dBm)) -> BB gain/2(P_IN_RSSI), RF Gain/1(Rx Pwr)
  RSSI Avg/1(avg) -> Capture & Convert/2(RSSI)
  RSSI/1 -> RSSI Avg/1(RSSI)
  Register1/1 -> Register2/1
  RF Gain/1(G_RF) -> Capture & Convert/1(G_RF), Register1/1

== system w2_warplab_agc/Gain Calc C ==
  I : Inport
  Q : Inport  Port=2
  IQ Valid : Inport  Port=3
  RSSI : Inport  Port=4
  BB gain : Subsystem
  Capture & Convert : Subsystem
  IQ Mag : Subsystem
  RF Gain : Subsystem
  RSSI Avg : Subsystem
  Register{1..4} (4 alike) : xbsIndex_r4/Register  init=0  rst=off  en=off  dbl_ovrd=off  block_type=register
  G_RF : Outport
  G_BB : Outport  Port=2
  wires:
  RF Gain/1(G_RF) -> Register1/1, Capture & Convert/1(G_RF)
  Register1/1 -> Register2/1
  RSSI/1 -> RSSI Avg/1(RSSI)
  RSSI Avg/1(avg) -> Capture & Convert/2(RSSI)
  Capture & Convert/1(Rx Pwr (dBm)) -> RF Gain/1(Rx Pwr), BB gain/2(P_IN_RSSI)
  Register3/1 -> Register4/1
  BB gain/1(G_BB) -> Register3/1
  RF Gain/2(G_RF_dB) -> BB gain/1(G_RF_dB)
  IQ Mag/1(IQ_dBv) -> BB gain/3(IQ_dBv)
  I/1 -> IQ Mag/1(I)
  Q/1 -> IQ Mag/2(Q)
  IQ Valid/1 -> IQ Mag/3(Valid)
  Register2/1 -> G_RF/1
  Register4/1 -> G_BB/1

== system w2_warplab_agc/Gain Calc D ==
  I : Inport
  Q : Inport  Port=2
  IQ Valid : Inport  Port=3
  RSSI : Inport  Port=4
  BB gain : Subsystem
  Capture & Convert : Subsystem
  IQ Mag : Subsystem
  RF Gain : Subsystem
  RSSI Avg : Subsystem
  Register{1..4} (4 alike) : xbsIndex_r4/Register  init=0  rst=off  en=off  dbl_ovrd=off  block_type=register
  G_RF : Outport
  G_BB : Outport  Port=2
  wires:
  Register4/1 -> G_BB/1
  Register2/1 -> G_RF/1
  IQ Valid/1 -> IQ Mag/3(Valid)
  Q/1 -> IQ Mag/2(Q)
  I/1 -> IQ Mag/1(I)
  IQ Mag/1(IQ_dBv) -> BB gain/3(IQ_dBv)
  RF Gain/2(G_RF_dB) -> BB gain/1(G_RF_dB)
  BB gain/1(G_BB) -> Register3/1
  Register3/1 -> Register4/1
  Capture & Convert/1(Rx Pwr (dBm)) -> BB gain/2(P_IN_RSSI), RF Gain/1(Rx Pwr)
  RSSI Avg/1(avg) -> Capture & Convert/2(RSSI)
  RSSI/1 -> RSSI Avg/1(RSSI)
  Register1/1 -> Register2/1
  RF Gain/1(G_RF) -> Capture & Convert/1(G_RF), Register1/1

== system w2_warplab_agc/IQ Outputs ==
  IQ Valid : Inport
  A I : Inport  Port=2
  A Q : Inport  Port=3
  B I : Inport  Port=4
  B Q : Inport  Port=5
  C I : Inport  Port=6
  C Q : Inport  Port=7
  D I : Inport  Port=8
  D Q : Inport  Port=9
  IQ_Valid_Out : xbsIndex_r4/Gateway Out  inherit_from_input=off  hdl_port=on  timing_constraint=None  locs_specified=off  LOCs={}  UseAsDAC=off  DACChannel='1'  block_type=gatewayout
  RFA_RX_I_OUT : xbsIndex_r4/Gateway Out  inherit_from_input=off  hdl_port=on  timing_constraint=None  locs_specified=off  LOCs={}  UseAsDAC=off  DACChannel='1'  block_type=gatewayout
  RFA_RX_Q_OUT : xbsIndex_r4/Gateway Out  inherit_from_input=off  hdl_port=on  timing_constraint=None  locs_specified=off  LOCs={}  UseAsDAC=off  DACChannel='1'  block_type=gatewayout
  RFB_RX_I_OUT : xbsIndex_r4/Gateway Out  inherit_from_input=off  hdl_port=on  timing_constraint=None  locs_specified=off  LOCs={}  UseAsDAC=off  DACChannel='1'  block_type=gatewayout
  RFB_RX_Q_OUT : xbsIndex_r4/Gateway Out  inherit_from_input=off  hdl_port=on  timing_constraint=None  locs_specified=off  LOCs={}  UseAsDAC=off  DACChannel='1'  block_type=gatewayout
  RFC_RX_I_OUT : xbsIndex_r4/Gateway Out  inherit_from_input=off  hdl_port=on  timing_constraint=None  locs_specified=off  LOCs={}  UseAsDAC=off  DACChannel='1'  block_type=gatewayout
  RFC_RX_Q_OUT : xbsIndex_r4/Gateway Out  inherit_from_input=off  hdl_port=on  timing_constraint=None  locs_specified=off  LOCs={}  UseAsDAC=off  DACChannel='1'  block_type=gatewayout
  RFD_RX_I_OUT : xbsIndex_r4/Gateway Out  inherit_from_input=off  hdl_port=on  timing_constraint=None  locs_specified=off  LOCs={}  UseAsDAC=off  DACChannel='1'  block_type=gatewayout
  RFD_RX_Q_OUT : xbsIndex_r4/Gateway Out  inherit_from_input=off  hdl_port=on  timing_constraint=None  locs_specified=off  LOCs={}  UseAsDAC=off  DACChannel='1'  block_type=gatewayout
  wires:
  A I/1 -> RFA_RX_I_OUT/1
  A Q/1 -> RFA_RX_Q_OUT/1
  IQ Valid/1 -> IQ_Valid_Out/1
  B I/1 -> RFB_RX_I_OUT/1
  B Q/1 -> RFB_RX_Q_OUT/1
  C I/1 -> RFC_RX_I_OUT/1
  C Q/1 -> RFC_RX_Q_OUT/1
  D I/1 -> RFD_RX_I_OUT/1
  D Q/1 -> RFD_RX_Q_OUT/1

== system w2_warplab_agc/RSSI Src ==
  Add : Sum
  Band-Limited White Noise : simulink/Sources/Band-Limited White Noise  SystemSampleTime=-1  Cov=200  Ts=1  seed=abs(ceil(1000*randn))
  Constant : Constant  Value=750
  Down Sample{,1..3} (4 alike) : xbsIndex_r4/Down Sample  sample_ratio=16  sample_phase="Last Value of Frame  (most efficient)"  en=off  latency=1  dbl_ovrd=off  block_type=dsamp
  RFA_RSSI : xbsIndex_r4/Gateway In  gui_display_data_type=Fixed-point  arith_type=Unsigned  n_bits=10  bin_pt=0  preci_type=Single  exp_width=8  frac_width=24  quantization="Round  (unbiased: +/- Inf)"  overflow=Saturate  period=1  dbl_ovrd=off  timing_constraint=None  locs_specified=off  LOCs={}  UseAsADC=off  ADCChannel='1'  inherit_from_input=off  hdl_port=on  block_type=gatewayin
  RFB_RSSI : xbsIndex_r4/Gateway In  gui_display_data_type=Fixed-point  arith_type=Unsigned  n_bits=10  bin_pt=0  preci_type=Single  exp_width=8  frac_width=24  quantization="Round  (unbiased: +/- Inf)"  overflow=Saturate  period=1  dbl_ovrd=off  timing_constraint=None  locs_specified=off  LOCs={}  UseAsADC=off  ADCChannel='1'  inherit_from_input=off  hdl_port=on  block_type=gatewayin
  RFC_RSSI : xbsIndex_r4/Gateway In  gui_display_data_type=Fixed-point  arith_type=Unsigned  n_bits=10  bin_pt=0  preci_type=Single  exp_width=8  frac_width=24  quantization="Round  (unbiased: +/- Inf)"  overflow=Saturate  period=1  dbl_ovrd=off  timing_constraint=None  locs_specified=off  LOCs={}  UseAsADC=off  ADCChannel='1'  inherit_from_input=off  hdl_port=on  block_type=gatewayin
  RFD_RSSI : xbsIndex_r4/Gateway In  gui_display_data_type=Fixed-point  arith_type=Unsigned  n_bits=10  bin_pt=0  preci_type=Single  exp_width=8  frac_width=24  quantization="Round  (unbiased: +/- Inf)"  overflow=Saturate  period=1  dbl_ovrd=off  timing_constraint=None  locs_specified=off  LOCs={}  UseAsADC=off  ADCChannel='1'  inherit_from_input=off  hdl_port=on  block_type=gatewayin
  Register{,1..3} (4 alike) : xbsIndex_r4/Register  init=0  rst=off  en=off  dbl_ovrd=off  block_type=register
  " RFA_RSSI" : Outport
  " RFB_RSSI" : Outport  Port=2
  " RFC_RSSI" : Outport  Port=3
  " RFD_RSSI" : Outport  Port=4
  wires:
  RFA_RSSI/1 -> Register/1
  Register/1 -> Down Sample/1
  Down Sample/1 -> " RFA_RSSI"/1
  Add/1 -> RFA_RSSI/1, RFB_RSSI/1, RFC_RSSI/1, RFD_RSSI/1
  Constant/1 -> Add/1
  Band-Limited White Noise/1 -> Add/2
  RFB_RSSI/1 -> Register1/1
  Register1/1 -> Down Sample1/1
  Down Sample1/1 -> " RFB_RSSI"/1
  RFC_RSSI/1 -> Register2/1
  RFD_RSSI/1 -> Register3/1
  Register2/1 -> Down Sample2/1
  Register3/1 -> Down Sample3/1
  Down Sample3/1 -> " RFD_RSSI"/1
  Down Sample2/1 -> " RFC_RSSI"/1
